simulink model "iWalker_dataHarvest"  (R2014a)
settings: Solver=ode3  StartTime=0.0  StopTime=10  FixedStep=0.01  RelTol=1e-3
InitFcn:
  | Ts=0.01
  | lid = LIDAR();
  | rob = DifferentialRobot();
  | rob.attachLidar(lid, [0.6,0,0]);
  | rob.dt = Ts;
  | ext = LandmarkExtractor();
  | ext.angularTolerance = 10.0;
  | map = LandmarkMap('test');
  | V = diag([0.005, 0.1*pi/180].^2);
  | P0 = diag([0.05, 0.05, 0.01].^2);
  | W = diag([0.05, 3*pi/180].^2);
  | ekf = EKFSLAM(rob, V, P0, 'map', map, 'estMap', true, 'W', W);
  | figure;
  | axis equal;
  | hold on;
  | whitebg([0 0 0]);
  | grid on;
  | 
  | pl = Plotter(gca);
libraries: iWalkerLib x1
settings Model: Creator=alumno  LastModifiedBy=Brian
settings DataIOCC: SignalLoggingSaveFormat=ModelDataLogs
settings OptimizationCC: ExpressionDepthLimit=2147483647  InitFltsAndDblsToZero=on
settings DebuggingCC: UnderspecifiedInitializationDetection=Classic  FcnCallInpInsideContextMsg=UseLocalSettings  StateNameClashWarn=warning
settings HardwareCC: TargetEndianess=LittleEndian  TargetHWDeviceType=MATLAB Host  ProdEqTarget=off
settings GRTTargetCC: CombineOutputUpdateFcns=off  GRTInterface=on

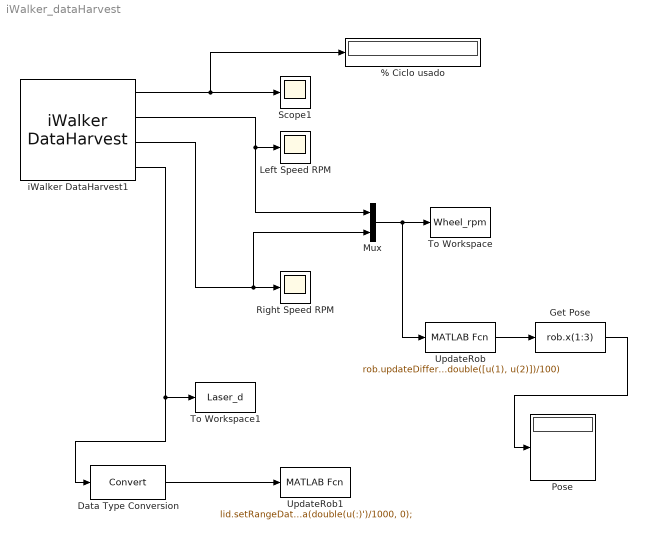
== system iWalker_dataHarvest ==
  % Ciclo usado : Display
      settings: Decimation=100
  Data Type Conversion : DataTypeConversion
  Get Pose : MATLABFcn  MATLABFcn=rob.x(1:3)  Output1D=off
  Left Speed RPM : Scope
      settings: TimeRange=10  YMin=-100  YMax=100
  Mux : Mux  Inputs=2
  Pose : Display
  Right Speed RPM : Scope
      settings: TimeRange=10  YMin=-100  YMax=100  SaveName=ScopeData2
  Scope1 : Scope
      settings: TimeRange=0.7489177489177488  YMin=0  YMax=250
  To Workspace : ToWorkspace  VariableName=Wheel_rpm  SaveFormat=Structure With Time  SampleTime=-1
  To Workspace1 : ToWorkspace  VariableName=Laser_d  SaveFormat=Structure With Time  SampleTime=-1
  UpdateRob : MATLABFcn  MATLABFcn=rob.updateDifferential(double([u(1), u(2)])/100)  Output1D=off
  UpdateRob1 : MATLABFcn  MATLABFcn=lid.setRangeData(double(u(:)')/1000, 0);  OutputDimensions=0  Output1D=off
  iWalker DataHarvest1 : iWalkerLib/iWalker DataHarvest
  wires:
  iWalker DataHarvest1/1 -> Scope1/1, % Ciclo usado/1
  iWalker DataHarvest1/2 -> Mux/1, Left Speed RPM/1
  iWalker DataHarvest1/3 -> Mux/2, Right Speed RPM/1
  Mux/1 -> UpdateRob/1, To Workspace/1
  iWalker DataHarvest1/4 -> Data Type Conversion/1, To Workspace1/1
  UpdateRob/1 -> Get Pose/1
  Get Pose/1 -> Pose/1
  Data Type Conversion/1 -> UpdateRob1/1
